simulink model "vehicle_parked_MIL"  (R2019a)
settings: Solver=FixedStepDiscrete  StartTime=0.0  StopTime=15  FixedStep=1  RelTol=1e-3
values from neighbouring files (symbols this model uses):
  Ignition = timeseries    [TT1_in.m]
undefined symbols (not defined in the file or in its folder): DN, Light, Lock
libraries: simulink x10
settings Model: Creator=vmadmin  LastModifiedBy=vmadmin
settings ConfigComp: CovMetricSettings=dcmw  CovHtmlReporting=on

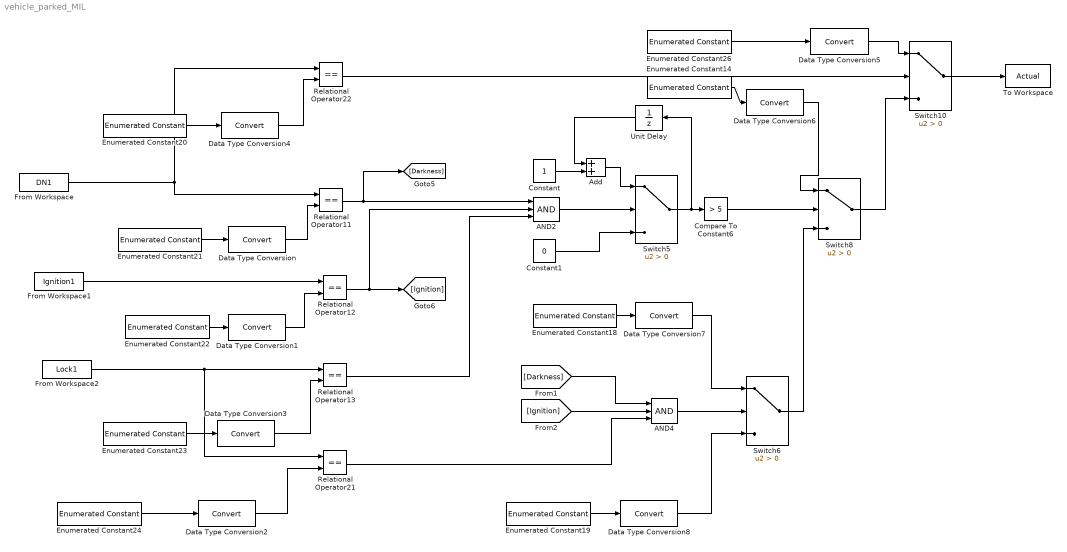
== system vehicle_parked_MIL ==
  AND2 : Logic  Inputs=3  AllPortsSameDT=off  OutDataTypeStr=boolean
  AND4 : Logic  Inputs=3  AllPortsSameDT=off  OutDataTypeStr=boolean
  Add : Sum
  Compare To Constant6 : simulink/Logic and Bit Operations/Compare To Constant  relop=>  const=5  OutDataTypeStr=boolean
  Constant : Constant
  Constant1 : Constant  Value=0
  Data Type Conversion{,1..8} (9 alike) : DataTypeConversion
  Enumerated Constant14 : simulink/Sources/Enumerated Constant  OutDataTypeStr=Enum: Light  Value=Light.Headlight_Off  SampleTime=inf
  Enumerated Constant18 : simulink/Sources/Enumerated Constant  OutDataTypeStr=Enum: Light  Value=Light.Low_Beam  SampleTime=inf
  Enumerated Constant19 : simulink/Sources/Enumerated Constant  OutDataTypeStr=Enum: Light  Value=Light.Low_Beam  SampleTime=inf
  Enumerated Constant20 : simulink/Sources/Enumerated Constant  OutDataTypeStr=Enum: DN  Value=DN.Day_Time  SampleTime=inf
  Enumerated Constant21 : simulink/Sources/Enumerated Constant  OutDataTypeStr=Enum: DN  Value=DN.Darkness  SampleTime=inf
  Enumerated Constant22 : simulink/Sources/Enumerated Constant  OutDataTypeStr=Enum: Ignition  Value=Ignition.Ignition_Off  SampleTime=inf
  Enumerated Constant23 : simulink/Sources/Enumerated Constant  OutDataTypeStr=Enum: Lock  Value=Lock.Vehicle_locked  SampleTime=inf
  Enumerated Constant24 : simulink/Sources/Enumerated Constant  OutDataTypeStr=Enum: Lock  Value=Lock.Vehicle_locked  SampleTime=inf
  Enumerated Constant26 : simulink/Sources/Enumerated Constant  OutDataTypeStr=Enum: Light  Value=Light.Headlight_Off  SampleTime=inf
  From Workspace : FromWorkspace  VariableName=DN1  SampleTime=0
  From Workspace1 : FromWorkspace  VariableName=Ignition1  SampleTime=0
  From Workspace2 : FromWorkspace  VariableName=Lock1  SampleTime=0
  Relational Operator{11..13,21..22} (5 alike) : RelationalOperator  Operator===  OutDataTypeStr=boolean  RndMeth=Simplest
  Switch{5..6,8,10} (4 alike) : Switch  Criteria=u2 > Threshold
  To Workspace : ToWorkspace  VariableName=Actual  SaveFormat=Timeseries  SampleTime=-1
  Unit Delay : UnitDelay  SampleTime=-1  HasFrameUpgradeWarning=on
  wires:
  Add/1 -> Switch5/1
  Switch5/1 -> Unit Delay/1, Compare To Constant6/1
  Enumerated Constant21/1 -> Data Type Conversion/1
  Enumerated Constant20/1 -> Data Type Conversion4/1
  Relational Operator22/1 -> Switch10/2
  From Workspace1/1 -> Relational Operator12/1
  [Ignition] -> AND4/2
  Constant/1 -> Add/2
  Relational Operator21/1 -> AND4/3
  AND2/1 -> Switch5/2
  Switch10/1 -> To Workspace/1
  Switch6/1 -> Switch8/3
  AND4/1 -> Switch6/2
  Enumerated Constant19/1 -> Data Type Conversion8/1
  Enumerated Constant18/1 -> Data Type Conversion7/1
  [Darkness] -> AND4/1
  Enumerated Constant23/1 -> Data Type Conversion3/1
  Constant1/1 -> Switch5/3
  From Workspace/1 -> Relational Operator11/1, Relational Operator22/1
  From Workspace2/1 -> Relational Operator13/1, Relational Operator21/1
  Enumerated Constant22/1 -> Data Type Conversion1/1
  Compare To Constant6/1 -> Switch8/2
  Enumerated Constant14/1 -> Data Type Conversion6/1
  Switch8/1 -> Switch10/3
  Relational Operator13/1 -> AND2/3
  Unit Delay/1 -> Add/1
  Relational Operator12/1 -> [Ignition], AND2/2
  Enumerated Constant24/1 -> Data Type Conversion2/1
  Enumerated Constant26/1 -> Data Type Conversion5/1
  Relational Operator11/1 -> [Darkness], AND2/1
  Data Type Conversion/1 -> Relational Operator11/2
  Data Type Conversion1/1 -> Relational Operator12/2
  Data Type Conversion3/1 -> Relational Operator13/2
  Data Type Conversion2/1 -> Relational Operator21/2
  Data Type Conversion4/1 -> Relational Operator22/2
  Data Type Conversion6/1 -> Switch8/1
  Data Type Conversion5/1 -> Switch10/1
  Data Type Conversion7/1 -> Switch6/1
  Data Type Conversion8/1 -> Switch6/3
